simulink model "supervision_simulation"  (Simulink 8.2)
settings: Solver=ode8  StartTime=0.0  StopTime=30  RelTol=1e-3
settings Model: Creator=petter  LastModifiedBy=petter
settings DataIOCC: SaveOutput=off  SaveTime=off
settings OptimizationCC: ExpressionDepthLimit=128
settings DebuggingCC: MultiTaskDSMMsg=warning  MultiTaskCondExecSysMsg=none  FcnCallInpInsideContextMsg=EnableAllAsError
settings RTWCC: IncludeERTFirstTime=on
settings GRTTargetCC: CombineOutputUpdateFcns=on  GRTInterface=off

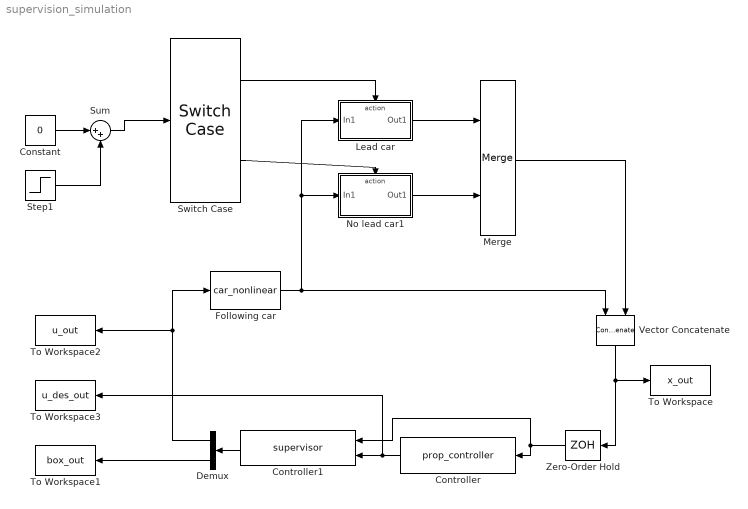
== system supervision_simulation ==
  Constant : Constant  Value=0
  Controller : M-S-Function  FunctionName=prop_controller
  Controller1 : M-S-Function  FunctionName=supervisor  Parameters=1,1
  Demux : Demux  Outputs=2
  Following car : M-S-Function  FunctionName=car_nonlinear  Parameters=25
  Lead car : Subsystem  TreatAsAtomicUnit=on
  Merge : Merge
  No lead car1 : Subsystem  TreatAsAtomicUnit=on
  Step1 : Step  Time=4  SampleTime=0
  Sum : Sum  Inputs=|++
  Switch Case : SwitchCase
  To Workspace : ToWorkspace  VariableName=x_out  SampleTime=-1  SaveFormat=Structure With Time
  To Workspace1 : ToWorkspace  VariableName=box_out  SampleTime=-1  SaveFormat=Structure With Time
  To Workspace2 : ToWorkspace  VariableName=u_out  SampleTime=-1  SaveFormat=Structure With Time
  To Workspace3 : ToWorkspace  VariableName=u_des_out  SampleTime=-1  SaveFormat=Structure With Time
  Vector Concatenate : Concatenate
  Zero-Order Hold : ZeroOrderHold  SampleTime=0.1
  wires:
  Demux/1 -> To Workspace2/1, Following car/1
  Zero-Order Hold/1 -> Controller1/1, Controller/1
  Merge/1 -> Vector Concatenate/2
  Vector Concatenate/1 -> Zero-Order Hold/1, To Workspace/1
  Controller1/1 -> Demux/1
  Controller/1 -> To Workspace3/1, Controller1/2
  Demux/2 -> To Workspace1/1
  Constant/1 -> Sum/1
  Lead car/1(Out1) -> Merge/1
  Switch Case/1 -> Lead car/Action
  Following car/1 -> Vector Concatenate/1, No lead car1/1(In1), Lead car/1(In1)
  Sum/1 -> Switch Case/1
  Switch Case/2 -> No lead car1/Action
  No lead car1/1(Out1) -> Merge/2
  Step1/1 -> Sum/2

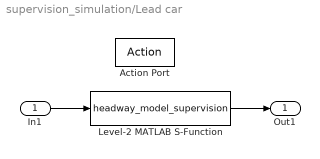
== system supervision_simulation/Lead car ==
  In1 : Inport
  Action Port : ActionPort  InitializeStates=reset  ActionType=case
  Level-2 MATLAB S-Function : M-S-Function  FunctionName=headway_model_supervision  Parameters=40, 15
  Out1 : Outport
  wires:
  In1/1 -> Level-2 MATLAB S-Function/1
  Level-2 MATLAB S-Function/1 -> Out1/1

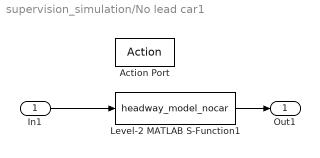
== system supervision_simulation/No lead car1 ==
  In1 : Inport
  Action Port : ActionPort  InitializeStates=reset  ActionType=default
  Level-2 MATLAB S-Function1 : M-S-Function  FunctionName=headway_model_nocar  Parameters=200.1
  Out1 : Outport
  wires:
  In1/1 -> Level-2 MATLAB S-Function1/1
  Level-2 MATLAB S-Function1/1 -> Out1/1
